simulink model "ES2_simulink"  (R2023b)
settings: Solver=VariableStepAuto  StartTime=0.0  StopTime=30.0  RelTol=1e-3
undefined symbols (not defined in the file or in its folder): fdesignblkfcn, gcbh
libraries: dspfdesign x5, vrlib x2
settings Model: NumberOfSteps=100  Creator=manu  LastModifiedBy=galvd

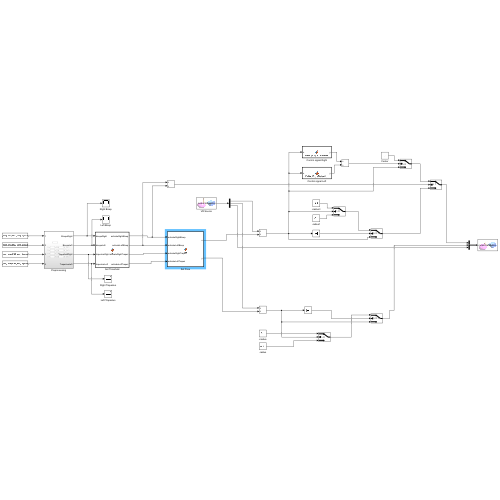
[thumbnail: Simulink's stored preview of the top-level diagram]
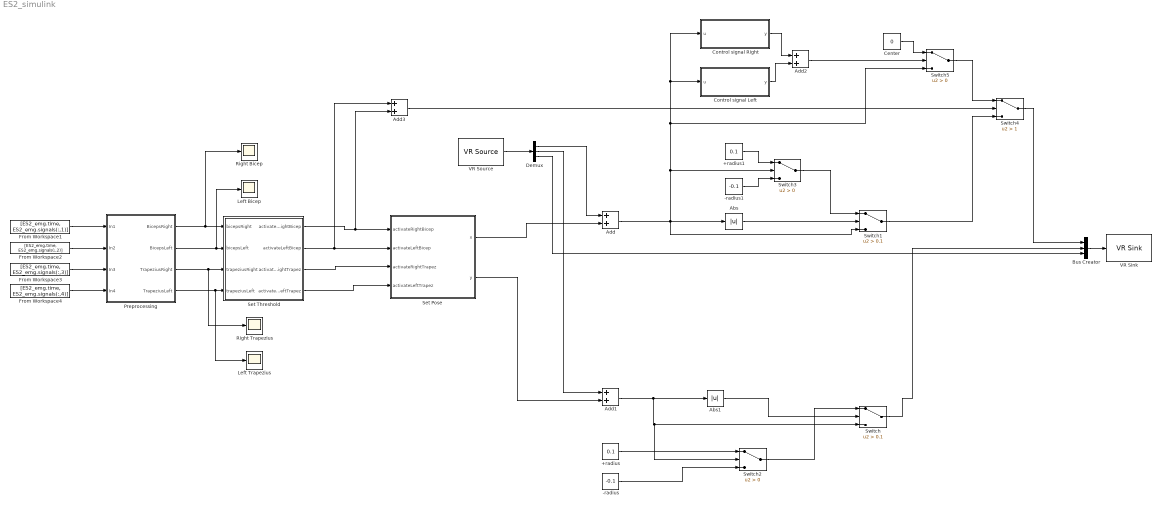
== system ES2_simulink ==
  +radius : Constant  Value=0.1
  +radius1 : Constant  Value=0.1
  -radius : Constant  Value=-0.1
  -radius1 : Constant  Value=-0.1
  Abs : Abs  SaturateOnIntegerOverflow=off
  Abs1 : Abs  SaturateOnIntegerOverflow=off
  Add{,1..3} (4 alike) : Sum
  Bus Creator : BusCreator  Inputs=3
  Center : Constant  Value=0
  Control signal Left : MATLAB Function  TreatAsAtomicUnit=on
  Control signal Right : MATLAB Function  TreatAsAtomicUnit=on
  Demux : Demux  Outputs=3
  From Workspace1 : FromWorkspace  VariableName=[ES2_emg.time, ES2_emg.signals(:,1)]  OutDataTypeStr=double  SampleTime=0.001
  From Workspace2 : FromWorkspace  VariableName=[ES2_emg.time, ES2_emg.signals(:,2)]  OutDataTypeStr=double  SampleTime=0.001
  From Workspace3 : FromWorkspace  VariableName=[ES2_emg.time, ES2_emg.signals(:,3)]  OutDataTypeStr=double  SampleTime=0.001
  From Workspace4 : FromWorkspace  VariableName=[ES2_emg.time, ES2_emg.signals(:,4)]  OutDataTypeStr=double  SampleTime=0.001
  Left Bicep : Scope
  Left Trapezius : Scope
  Preprocessing : Subsystem
  Right Bicep : Scope
  Right Trapezius : Scope
  Set Pose : MATLAB Function  TreatAsAtomicUnit=on
  Set Threshold : MATLAB Function  TreatAsAtomicUnit=on
  Switch : Switch  Criteria=u2 > Threshold  Threshold=0.1  SaturateOnIntegerOverflow=off  InputSameDT=off
  Switch1 : Switch  Criteria=u2 > Threshold  Threshold=0.1  SaturateOnIntegerOverflow=off  InputSameDT=off
  Switch2 : Switch  Criteria=u2 > Threshold  SaturateOnIntegerOverflow=off  InputSameDT=off
  Switch3 : Switch  Criteria=u2 > Threshold  SaturateOnIntegerOverflow=off  InputSameDT=off
  Switch4 : Switch  Criteria=u2 > Threshold  Threshold=1  SaturateOnIntegerOverflow=off  InputSameDT=off
  Switch5 : Switch  Criteria=u2 > Threshold  SaturateOnIntegerOverflow=off  InputSameDT=off
  VR Sink : vrlib/VR Sink  InstantiateOnLoad=on  SampleTime=0.1  ViewEnable=on  RemoteChange=off  RemoteView=off  FieldsWritten=cursor.translation.3.1.1.double  WorldFileName=8_palline_color.wrl  AutoView=off  VideoDimensions=[]  AllowVariableSize=off
  VR Source : vrlib/VR Source  InstantiateOnLoad=on  SampleTime=0.1  ViewEnable=on  RemoteChange=off  RemoteView=off  FieldsRead=cursor.translation.1.3.1.double  WorldFileName=8_palline_color.wrl  AutoView=off  VideoDimensions=[]  AllowVariableSize=off  FigureProperties="{'Position', 'Name', 'Viewpoint', 'CameraBound', 'CameraDirection', 'CameraPosition', 'CameraUpVector', 'ZoomFactor', 'Antialiasing', 'Headlight', 'Lighting', 'NavPanel', 'Sound', 'StatusBar', 'Stereo3D', 'Stereo3DCameraOffset', 'Stereo3DHIT', 'ToolBar', 'Textures', 'Transparency', 'Triad', 'Wireframe', 'NavZones', 'NavMode', 'NavSpeed', 'CaptureFileFormat', 'CaptureFileName', 'Record2DCompressMethod', 'Record2DCompressQuality', 'Record2D', 'Record2DFileName', 'Record2DFPS'; [4.5500000000000000e+02   2.8900000000000000e+02   5.7600000000000000e+02   3.5000000000000000e+02], '', '_untitled_1', 'on', [0.0000000000000000e+00   0.0000000000000000e+00  -1.0000000000000000e+00], [0.0000000000000000e+00   0.0000000000000000e+00   0.0000000000000000e+00], [0.0000000000000000e+00   1.0000000000000000e+00   0.0000000000000000e+00], [1.0000000000000000e+00], 'on', 'on', 'on', 'halfbar', 'on', 'on', 'off', [1.0000000149011612e-01], [0.0000000000000000e+00], 'on', 'on', 'on', 'none', 'off', 'off', 'fly', 'normal', 'tif', '%f_anim_%n.tif', 'auto', [7.5000000000000000e+01], 'off', '%f_anim_%n.avi', 'auto'}"
  wires:
  From Workspace1/1 -> Preprocessing/1(In1)
  From Workspace2/1 -> Preprocessing/2(In2)
  From Workspace3/1 -> Preprocessing/3(In3)
  From Workspace4/1 -> Preprocessing/4(In4)
  VR Source/1 -> Demux/1
  Bus Creator/1 -> VR Sink/1
  Set Pose/1(x) -> Add/2
  Set Pose/2(y) -> Add1/2
  Demux/1 -> Add/1
  Demux/2 -> Add1/1
  Set Threshold/2(activateLeftBicep) -> Add3/1, Set Pose/2(activateLeftBicep)
  Set Threshold/3(activateRightTrapez) -> Set Pose/3(activateRightTrapez)
  Set Threshold/4(activateLeftTrapez) -> Set Pose/4(activateLeftTrapez)
  Preprocessing/3(TrapeziusRight) -> Right Trapezius/1, Set Threshold/3(trapeziusRight)
  Preprocessing/4(TrapeziusLeft) -> Left Trapezius/1, Set Threshold/4(trapeziusLeft)
  Add1/1 -> Switch2/2, Switch/3, Abs1/1
  Demux/3 -> Bus Creator/3
  Preprocessing/1(BicepsRight) -> Right Bicep/1, Set Threshold/1(bicepsRight)
  Preprocessing/2(BicepsLeft) -> Left Bicep/1, Set Threshold/2(bicepsLeft)
  +radius/1 -> Switch2/1
  Switch/1 -> Bus Creator/2
  Abs/1 -> Switch1/2
  Abs1/1 -> Switch/2
  -radius/1 -> Switch2/3
  Switch2/1 -> Switch/1
  +radius1/1 -> Switch3/1
  -radius1/1 -> Switch3/3
  Switch3/1 -> Switch1/1
  Switch4/1 -> Bus Creator/1
  Switch1/1 -> Switch4/3
  Add/1 -> Switch5/3, Control signal Right/1(u), Control signal Left/1(u), Switch3/2, Switch1/3, Abs/1
  Control signal Right/1(y) -> Add2/1
  Control signal Left/1(y) -> Add2/2
  Add2/1 -> Switch5/2
  Center/1 -> Switch5/1
  Switch5/1 -> Switch4/1
  Set Threshold/1(activateRightBicep) -> Add3/2, Set Pose/1(activateRightBicep)
  Add3/1 -> Switch4/2

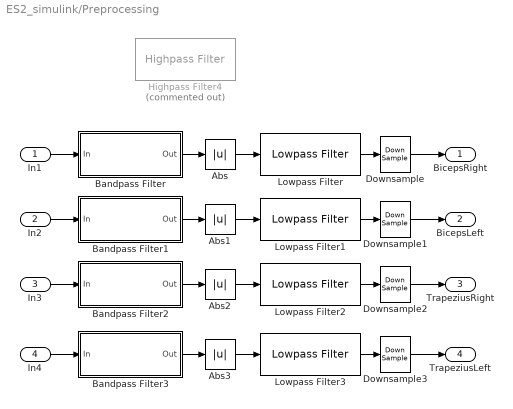
== system ES2_simulink/Preprocessing ==
  In1 : Inport
  In2 : Inport  Port=2
  In3 : Inport  Port=3
  In4 : Inport  Port=4
  Abs{,1..3} (4 alike) : Abs  SaturateOnIntegerOverflow=off
  Bandpass Filter : Subsystem  DialogController=fdesignblkfcn  InitFcn=fdesignblkfcn(gcbh, {'InitFcn'});  mask(Bandpass Filter){}
      mask help: dsp:DSPFilterDesignBlockDialog:BandpassFdesign_MaskDesc
      settings: CopyFcn=fdesignblkfcn(gcbh, {'CopyFcn'});
      mask Help: helpview(mapfilelocation('dsp'), 'dspbandpassfilter');
      mask Display: disp('Bandpass');
  Bandpass Filter1 : Subsystem  DialogController=fdesignblkfcn  InitFcn=fdesignblkfcn(gcbh, {'InitFcn'});  mask(Bandpass Filter){}
      mask help: dsp:DSPFilterDesignBlockDialog:BandpassFdesign_MaskDesc
      settings: CopyFcn=fdesignblkfcn(gcbh, {'CopyFcn'});
      mask Help: helpview(mapfilelocation('dsp'), 'dspbandpassfilter');
      mask Display: disp('Bandpass');
  Bandpass Filter2 : Subsystem  DialogController=fdesignblkfcn  InitFcn=fdesignblkfcn(gcbh, {'InitFcn'});  mask(Bandpass Filter){}
      mask help: dsp:DSPFilterDesignBlockDialog:BandpassFdesign_MaskDesc
      settings: CopyFcn=fdesignblkfcn(gcbh, {'CopyFcn'});
      mask Help: helpview(mapfilelocation('dsp'), 'dspbandpassfilter');
      mask Display: disp('Bandpass');
  Bandpass Filter3 : Subsystem  DialogController=fdesignblkfcn  InitFcn=fdesignblkfcn(gcbh, {'InitFcn'});  mask(Bandpass Filter){}
      mask help: dsp:DSPFilterDesignBlockDialog:BandpassFdesign_MaskDesc
      settings: CopyFcn=fdesignblkfcn(gcbh, {'CopyFcn'});
      mask Help: helpview(mapfilelocation('dsp'), 'dspbandpassfilter');
      mask Display: disp('Bandpass');
  Downsample{,1..3} (4 alike) : DownSample  N=4  RateOptions=Allow multirate processing
  Highpass Filter4 : dspfdesign/Highpass Filter  Commented=on  FilterType=FIR  DesignForMinimumOrder=on  FilterOrder=50  StopbandFrequency=30  PassbandFrequency=450  StopbandAttenuation=80  PassbandRipple=0.1  SampleRate=44100  SimulateUsing=Interpreted execution  roundingMode=Floor  coeffsDataTypeStr=fixdt(1,16)
  Lowpass Filter{,1..3} (4 alike) : dspfdesign/Lowpass Filter  FilterType=FIR  DesignForMinimumOrder=on  FilterOrder=50  PassbandFrequency=3  StopbandFrequency=6  PassbandRipple=0.1  StopbandAttenuation=80  SampleRateMode=Specify on dialog  SampleRate=1000  SimulateUsing=Interpreted execution  roundingMode=Floor  coeffsDataTypeStr=fixdt(1,16)
  BicepsRight : Outport
  BicepsLeft : Outport  Port=2
  TrapeziusRight : Outport  Port=3
  TrapeziusLeft : Outport  Port=4
  wires:
  Lowpass Filter2/1 -> Downsample2/1
  Bandpass Filter2/1(Out) -> Abs2/1
  Abs1/1 -> Lowpass Filter1/1
  Abs3/1 -> Lowpass Filter3/1
  Abs/1 -> Lowpass Filter/1
  Bandpass Filter3/1(Out) -> Abs3/1
  In4/1 -> Bandpass Filter3/1(In)
  In1/1 -> Bandpass Filter/1(In)
  Bandpass Filter/1(Out) -> Abs/1
  Bandpass Filter1/1(Out) -> Abs1/1
  Abs2/1 -> Lowpass Filter2/1
  Lowpass Filter1/1 -> Downsample1/1
  Downsample/1 -> BicepsRight/1
  Lowpass Filter3/1 -> Downsample3/1
  Lowpass Filter/1 -> Downsample/1
  Downsample3/1 -> TrapeziusLeft/1
  Downsample1/1 -> BicepsLeft/1
  In3/1 -> Bandpass Filter2/1(In)
  In2/1 -> Bandpass Filter1/1(In)
  Downsample2/1 -> TrapeziusRight/1

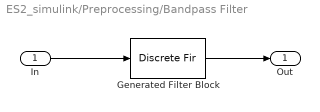
== system ES2_simulink/Preprocessing/Bandpass Filter ==
  In : Inport
  Generated Filter Block : DiscreteFir  Tag=BlockMethodSubSystem  Coefficients=[8.09984662039171167e-19 6.39138873735445952e-05 -0.000529985360713195602 0.000163049509978640958 -0.00106873656065133355 0.000138454107623771778 -0.00150740219393306354 -0.000146171169312381939 -0.00164491285071874664 -0.000803831165663842096 -0.00127002939103642264 -0.00179475969145176406 -0.000313202715390952153 -0.00280047053638836797 0.00102378750565708626 -0.00320898606072516192 0.00226847122552957785 -0.00229118992766688115 0.00286273128519679053 0.000444283590646493102 0.00248061645378650983 0.00484772649949967091 0.0013231555973298554 0.00988516690279817554 0.000195375038696813459 0.0137475146561206515 0.000235578061564314939 0.0143783789118079978 0.00232373851233996093 0.0102932854869860792 0.00637980828249819481 0.0013872101835551594 0.0108821641584975915 -0.0106388069047137126 0.0129164407258158982 -0.0225052497171089536 0.00888838159476280226 -0.0302697542973048087 -0.00424164083303872359 -0.0306714306083059364 -0.0276065409272709811 -0.022423923961180349 -0.0594922495550082378 -0.00693651358874992994 -0.0952531612511480497 0.0118816213758879876 -0.128243809353299015 0.0287429432612043914 -0.151547652016043505 0.0386729267839347052 0.839787881504184819 0.0386729267839347052 -0.151547652016043505 0.0287429432612043914 -0.128243809353299015 0.0118816213758879876 -0.0952531612511480497 -0.00693651358874992994 -0.0594922495550082378 -0.022423923961180349 -0.0276065409272709811 -0.0306714306083059364 -0.00424164083303872359 -0.0302697542973048087 0.00888838159476280226 -0.0225052497171089536 0.0129164407258158982 -0.0106388069047137126 0.0108821641584975915 0.0013872101835551594 0.00637980828249819481 0.0102932854869860792 0.00232373851233996093 0.0143783789118079978 0.000235578061564314939 0.0137475146561206515 0.000195375038696813459 0.00988516690279817554 0.0013231555973298554 0.00484772649949967091 0.00248061645378650983 0.000444283590646493102 0.00286273128519679053 -0.00229118992766688115 0.00226847122552957785 -0.00320898606072516192 0.00102378750565708626 -0.00280047053638836797 -0.000313202715390952153 -0.00179475969145176406 -0.00127002939103642264 -0.000803831165663842096 -0.00164491285071874664 -0.000146171169312381939 -0.00150740219393306354 0.000138454107623771778 -0.00106873656065133355 0.000163049509978640958 -0.000529985360713195602 6.39138873735445952e-05 8.09984662039171167e-19]  InputProcessing=Columns as channels (frame based)
  Out : Outport  VectorParamsAs1DForOutWhenUnconnected=off
  wires:
  In/1 -> Generated Filter Block/1
  Generated Filter Block/1 -> Out/1

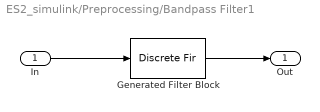
== system ES2_simulink/Preprocessing/Bandpass Filter1 ==
  In : Inport
  Generated Filter Block : DiscreteFir  Tag=BlockMethodSubSystem  Coefficients=[8.09984662039171167e-19 6.39138873735445952e-05 -0.000529985360713195602 0.000163049509978640958 -0.00106873656065133355 0.000138454107623771778 -0.00150740219393306354 -0.000146171169312381939 -0.00164491285071874664 -0.000803831165663842096 -0.00127002939103642264 -0.00179475969145176406 -0.000313202715390952153 -0.00280047053638836797 0.00102378750565708626 -0.00320898606072516192 0.00226847122552957785 -0.00229118992766688115 0.00286273128519679053 0.000444283590646493102 0.00248061645378650983 0.00484772649949967091 0.0013231555973298554 0.00988516690279817554 0.000195375038696813459 0.0137475146561206515 0.000235578061564314939 0.0143783789118079978 0.00232373851233996093 0.0102932854869860792 0.00637980828249819481 0.0013872101835551594 0.0108821641584975915 -0.0106388069047137126 0.0129164407258158982 -0.0225052497171089536 0.00888838159476280226 -0.0302697542973048087 -0.00424164083303872359 -0.0306714306083059364 -0.0276065409272709811 -0.022423923961180349 -0.0594922495550082378 -0.00693651358874992994 -0.0952531612511480497 0.0118816213758879876 -0.128243809353299015 0.0287429432612043914 -0.151547652016043505 0.0386729267839347052 0.839787881504184819 0.0386729267839347052 -0.151547652016043505 0.0287429432612043914 -0.128243809353299015 0.0118816213758879876 -0.0952531612511480497 -0.00693651358874992994 -0.0594922495550082378 -0.022423923961180349 -0.0276065409272709811 -0.0306714306083059364 -0.00424164083303872359 -0.0302697542973048087 0.00888838159476280226 -0.0225052497171089536 0.0129164407258158982 -0.0106388069047137126 0.0108821641584975915 0.0013872101835551594 0.00637980828249819481 0.0102932854869860792 0.00232373851233996093 0.0143783789118079978 0.000235578061564314939 0.0137475146561206515 0.000195375038696813459 0.00988516690279817554 0.0013231555973298554 0.00484772649949967091 0.00248061645378650983 0.000444283590646493102 0.00286273128519679053 -0.00229118992766688115 0.00226847122552957785 -0.00320898606072516192 0.00102378750565708626 -0.00280047053638836797 -0.000313202715390952153 -0.00179475969145176406 -0.00127002939103642264 -0.000803831165663842096 -0.00164491285071874664 -0.000146171169312381939 -0.00150740219393306354 0.000138454107623771778 -0.00106873656065133355 0.000163049509978640958 -0.000529985360713195602 6.39138873735445952e-05 8.09984662039171167e-19]  InputProcessing=Columns as channels (frame based)
  Out : Outport  VectorParamsAs1DForOutWhenUnconnected=off
  wires:
  In/1 -> Generated Filter Block/1
  Generated Filter Block/1 -> Out/1

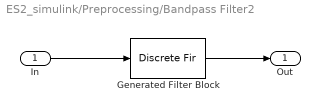
== system ES2_simulink/Preprocessing/Bandpass Filter2 ==
  In : Inport
  Generated Filter Block : DiscreteFir  Tag=BlockMethodSubSystem  Coefficients=[8.09984662039171167e-19 6.39138873735445952e-05 -0.000529985360713195602 0.000163049509978640958 -0.00106873656065133355 0.000138454107623771778 -0.00150740219393306354 -0.000146171169312381939 -0.00164491285071874664 -0.000803831165663842096 -0.00127002939103642264 -0.00179475969145176406 -0.000313202715390952153 -0.00280047053638836797 0.00102378750565708626 -0.00320898606072516192 0.00226847122552957785 -0.00229118992766688115 0.00286273128519679053 0.000444283590646493102 0.00248061645378650983 0.00484772649949967091 0.0013231555973298554 0.00988516690279817554 0.000195375038696813459 0.0137475146561206515 0.000235578061564314939 0.0143783789118079978 0.00232373851233996093 0.0102932854869860792 0.00637980828249819481 0.0013872101835551594 0.0108821641584975915 -0.0106388069047137126 0.0129164407258158982 -0.0225052497171089536 0.00888838159476280226 -0.0302697542973048087 -0.00424164083303872359 -0.0306714306083059364 -0.0276065409272709811 -0.022423923961180349 -0.0594922495550082378 -0.00693651358874992994 -0.0952531612511480497 0.0118816213758879876 -0.128243809353299015 0.0287429432612043914 -0.151547652016043505 0.0386729267839347052 0.839787881504184819 0.0386729267839347052 -0.151547652016043505 0.0287429432612043914 -0.128243809353299015 0.0118816213758879876 -0.0952531612511480497 -0.00693651358874992994 -0.0594922495550082378 -0.022423923961180349 -0.0276065409272709811 -0.0306714306083059364 -0.00424164083303872359 -0.0302697542973048087 0.00888838159476280226 -0.0225052497171089536 0.0129164407258158982 -0.0106388069047137126 0.0108821641584975915 0.0013872101835551594 0.00637980828249819481 0.0102932854869860792 0.00232373851233996093 0.0143783789118079978 0.000235578061564314939 0.0137475146561206515 0.000195375038696813459 0.00988516690279817554 0.0013231555973298554 0.00484772649949967091 0.00248061645378650983 0.000444283590646493102 0.00286273128519679053 -0.00229118992766688115 0.00226847122552957785 -0.00320898606072516192 0.00102378750565708626 -0.00280047053638836797 -0.000313202715390952153 -0.00179475969145176406 -0.00127002939103642264 -0.000803831165663842096 -0.00164491285071874664 -0.000146171169312381939 -0.00150740219393306354 0.000138454107623771778 -0.00106873656065133355 0.000163049509978640958 -0.000529985360713195602 6.39138873735445952e-05 8.09984662039171167e-19]  InputProcessing=Columns as channels (frame based)
  Out : Outport  VectorParamsAs1DForOutWhenUnconnected=off
  wires:
  In/1 -> Generated Filter Block/1
  Generated Filter Block/1 -> Out/1

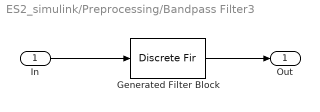
== system ES2_simulink/Preprocessing/Bandpass Filter3 ==
  In : Inport
  Generated Filter Block : DiscreteFir  Tag=BlockMethodSubSystem  Coefficients=[8.09984662039171167e-19 6.39138873735445952e-05 -0.000529985360713195602 0.000163049509978640958 -0.00106873656065133355 0.000138454107623771778 -0.00150740219393306354 -0.000146171169312381939 -0.00164491285071874664 -0.000803831165663842096 -0.00127002939103642264 -0.00179475969145176406 -0.000313202715390952153 -0.00280047053638836797 0.00102378750565708626 -0.00320898606072516192 0.00226847122552957785 -0.00229118992766688115 0.00286273128519679053 0.000444283590646493102 0.00248061645378650983 0.00484772649949967091 0.0013231555973298554 0.00988516690279817554 0.000195375038696813459 0.0137475146561206515 0.000235578061564314939 0.0143783789118079978 0.00232373851233996093 0.0102932854869860792 0.00637980828249819481 0.0013872101835551594 0.0108821641584975915 -0.0106388069047137126 0.0129164407258158982 -0.0225052497171089536 0.00888838159476280226 -0.0302697542973048087 -0.00424164083303872359 -0.0306714306083059364 -0.0276065409272709811 -0.022423923961180349 -0.0594922495550082378 -0.00693651358874992994 -0.0952531612511480497 0.0118816213758879876 -0.128243809353299015 0.0287429432612043914 -0.151547652016043505 0.0386729267839347052 0.839787881504184819 0.0386729267839347052 -0.151547652016043505 0.0287429432612043914 -0.128243809353299015 0.0118816213758879876 -0.0952531612511480497 -0.00693651358874992994 -0.0594922495550082378 -0.022423923961180349 -0.0276065409272709811 -0.0306714306083059364 -0.00424164083303872359 -0.0302697542973048087 0.00888838159476280226 -0.0225052497171089536 0.0129164407258158982 -0.0106388069047137126 0.0108821641584975915 0.0013872101835551594 0.00637980828249819481 0.0102932854869860792 0.00232373851233996093 0.0143783789118079978 0.000235578061564314939 0.0137475146561206515 0.000195375038696813459 0.00988516690279817554 0.0013231555973298554 0.00484772649949967091 0.00248061645378650983 0.000444283590646493102 0.00286273128519679053 -0.00229118992766688115 0.00226847122552957785 -0.00320898606072516192 0.00102378750565708626 -0.00280047053638836797 -0.000313202715390952153 -0.00179475969145176406 -0.00127002939103642264 -0.000803831165663842096 -0.00164491285071874664 -0.000146171169312381939 -0.00150740219393306354 0.000138454107623771778 -0.00106873656065133355 0.000163049509978640958 -0.000529985360713195602 6.39138873735445952e-05 8.09984662039171167e-19]  InputProcessing=Columns as channels (frame based)
  Out : Outport  VectorParamsAs1DForOutWhenUnconnected=off
  wires:
  In/1 -> Generated Filter Block/1
  Generated Filter Block/1 -> Out/1

== matlab function ES2_simulink/Set Threshold ==
  data: bicepsRight input; activateRightBicep output; activateLeftBicep output; activateRightTrapez output; activateLeftTrapez output; bicepsLeft input; trapeziusRight input; trapeziusLeft input
function [activateRightBicep, activateLeftBicep, activateRightTrapez, activateLeftTrapez] = fcn(bicepsRight, bicepsLeft, trapeziusRight, trapeziusLeft)
    persistent previousValue;
    persistent movement;

    if isempty(movement)
        movement = 1;
    end

    activateRightBicep = 0; 
    activateLeftBicep = 0;
    activateRightTrapez = 0;
    activateLeftTrapez = 0;

    if (movement == 1 && bicepsRight >= 0.16)
        movement = 2;
        previousValue = bicepsRight;
    end
    if (movement == 2 && bicepsRight <= 0.04)
        movement = 1;
        previousValue = bicepsRight;
    end

    if (bicepsRight > 0.04 && bicepsRight < 0.16)
        if movement == 1 % here we are moving to the ball
            if isempty(previousValue)
                previousValue = bicepsRight;
            else
                if bicepsRight > previousValue
                    activateRightBicep = 1;
                    previousValue = bicepsRight;
                end 
            end
        end
        if movement == 2 % here we are moving to the center
            if isempty(previousValue)
                previousValue = bicepsRight;
            else
                if bicepsRight < previousValue
                    activateRightBicep = 2;
                    previousValue = bicepsRight;
                end 
            end
        end   

  %  elseif bicepsLeft > 0.05
  %      activateLeftBicep = 1;
  % elseif trapeziusRight > 0.09
  %     activateRightTrapez = 1;
  % elseif trapeziusLeft > 0.04
  %     activateLeftTrapez = 1;
    end
            
end

== matlab function ES2_simulink/Set Pose ==
  data: activateRightBicep input; activateLeftBicep input; activateRightTrapez input; activateLeftTrapez input; x output; y output
function [x, y] = fcn(activateRightBicep,activateLeftBicep, activateRightTrapez, activateLeftTrapez)
    x = 0;
    y = 0;

    if activateRightBicep == 1
        x =  0.03;
    elseif activateRightBicep == 2
        x = -0.05;
    elseif activateLeftBicep == 1
        x = -0.0028;
    elseif activateRightTrapez == 1
        y =  0.009;
    elseif activateLeftTrapez == 1
        y = -0.0091;
    end
          
end

== matlab function ES2_simulink/Control signal Right ==
  data: u input; y output
function y = FallingEdgeDetection(u)
    persistent previousValue; 
    
    if isempty(previousValue)
        previousValue = u;
    end
    
    % Control if there is a signal change
    if (u < 0 && previousValue >= 0)
        y = 1;  % OK change signal
    else
        y = 0;  % NO change
    end

    previousValue = u;
end

== matlab function ES2_simulink/Control signal Left ==
  data: u input; y output
function y = FallingEdgeDetection(u)
    persistent previousValue; 
    
    if isempty(previousValue)
        previousValue = u;
    end
    
    % Control if there is a signal change
    if (u > 0 && previousValue <= 0)
        y = 1;  % OK change signal
    else
        y = 0;  % NO change
    end

    previousValue = u;
end
